simulink model "FM1"  (Simulink 7.0)
settings: Solver=ode45  StartTime=0.0  StopTime=1  RelTol=1e-3
libraries: simulink x2
settings Model: Creator=Antonio  LastModifiedBy=Antonio

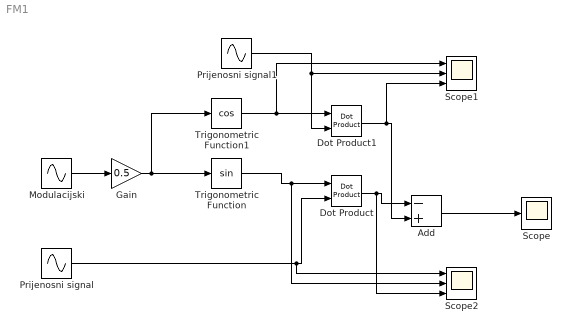
== system FM1 ==
  Add : Sum  Inputs=-+  OutDataType=sfix(16)  OutScaling=2^-10
  Dot Product : simulink/Math Operations/Dot Product  InputSameDT=on  OutDataType=sfix(16)  OutScaling=2^-10  DoSatur=off
  Dot Product1 : simulink/Math Operations/Dot Product  InputSameDT=on  OutDataType=sfix(16)  OutScaling=2^-10  DoSatur=off
  Gain : Gain  Gain=0.5  ParameterDataType=sfix(16)  ParameterScaling=2^0  OutDataType=sfix(16)  OutScaling=2^0
  Modulacijski : Sin  Frequency=2*pi*1000  SampleTime=1/100000
  Prijenosni signal : Sin  Frequency=2*pi*5000  Samples=100  SampleTime=1/100000
  Prijenosni signal1 : Sin  Frequency=2*pi*5000  Phase=pi/2  Samples=100  SampleTime=1/100000
  Scope : Scope
  Scope1 : Scope  NumInputPorts=3
      settings: YMin=-5~-5~-5  YMax=5~5~5
  Scope2 : Scope  NumInputPorts=3
      settings: YMin=-5~-5~-5  YMax=5~5~5  SaveName=ScopeData2
  Trigonometric Function : Trigonometry
  Trigonometric Function1 : Trigonometry  Operator=cos
  wires:
  Modulacijski/1 -> Gain/1
  Gain/1 -> Trigonometric Function/1, Trigonometric Function1/1
  Trigonometric Function/1 -> Dot Product/1, Scope2/2
  Prijenosni signal/1 -> Dot Product/2, Scope2/1
  Trigonometric Function1/1 -> Dot Product1/1, Scope1/1
  Dot Product/1 -> Add/1, Scope2/3
  Prijenosni signal1/1 -> Dot Product1/2, Scope1/2
  Dot Product1/1 -> Add/2, Scope1/3
  Add/1 -> Scope/1
